simulink model "HybridVehicle"  (R2020b)
settings: Solver=ode23tb  StartTime=0.0  StopTime=1800  RelTol=1e-3
model workspace (MAT data in the model file):
  DownShiftSpeeds = [11.05  11.05  11.05  11.05  11.05  11.05  11.05  11.05  11.05  11.05  11.05  11.05  19.55  25.5  31.45  35.7  35.7; 18.7  18.7  18.7  18.7  19.125  20.48636  21.33636  23.375  27.28636  30.26136  33.827365  38.76136  46.072635  56.1  64.6  73.1  73.1; 28.9  28.9  28.9  28.9  28.9  30.51364  34.51136  41.56364  47.68636  53.377365  58.477365  65.622635  73.525  81.26136  88.48636  115.6  115.6; 38.675  38.675  38.675  38.675  39.43864  42.41364  47.68636  56.43864  65.11136  72.927365  80.497635  90.01364  100.81136  110.672635  122.4  153  153; 51.425  51.425  51.425  51.425  51.76364  55.077365  62.38864  72.422635  83.3  102  136  425  425  425  425  425  425]
  I = 0.25
  Kbr = 1000000
  MGUMaxPower = 50000
  P = 15
  PedalPositions = [0 6.2485 12.4969 18.7454 24.9939 31.2424 37.4908 43.7393 49.9878 56.2363 62.4847 68.7332 74.9817 81.2302 87.4786 93.7271 99.9756]
  SOCmax = 99
  TrqICMax = 175
  TrqMGUMax = 150
  TrqMax = 325
  UpShiftSpeeds = [12.75  12.75  12.75  12.75  12.75  12.75  15.552365  17.08636  18.7  20.227365  23.46136  27.625  31.702365  36.63636  42.5  42.5  42.5; 20.997635  20.997635  20.997635  20.997635  21.927365  24.902365  28.727365  31.78864  35.275  39.697635  46.41136  51.85  59.672635  67.48864  78.2  78.2  78.2; 31.45  31.45  31.45  31.45  34.172635  41.052365  47.175  52.952365  59.5  68  76.5  85  93.5  106.25  119.85  119.85  119.85; 42.16136  42.16136  42.16136  43.947635  47.002365  54.31364  63.325  71.227365  79.222635  88.06136  98.852365  109.052365  118.402365  128.86136  157.25  157.25  157.25; 55.58864  55.58864  55.58864  58.052365  61.53864  72.077365  85.51136  96.81364  255  255  255  255  255  255  255  255  255]
  axle_b = 10
  axle_k = 5000
  bevAxle_wc = 400
  bevNp = 2
  bevNs = 30
  brkTrqMGU = 150
  brkTrqMax = 700
  convAxle_wc = 500
  diffRatio = 3.4
  diffRatio1 = 3.4
  driveshaft_b = 10
  driveshaft_k = 2500
  driveshaft_wc = 500
  engineSpeedPoints_rpm = [750 1053.57142857 1357.14285714 1660.71428571 1964.28571429 2267.85714286 2571.42857143 2875 3178.57142857 3482.14285714 3785.71428571 4089.28571429 4392.85714286 4696.42857143 5000]
  engineTorqueMap_Nm = [-13.6738264269 15.0034460821 26.4289521305 37.8539339756 49.2854604964 60.7146317399 72.0173711595 77.7345012802 77.7345012802 77.7345012802 77.7345012802 77.7345012802 ... (240 elements, 16x15)]
  engineTorquePoints_Nm = [0 15 26.4285714286 37.8571428571 49.2857142857 60.7142857143 72.1428571429 83.5714285714 95 106.428571429 117.857142857 129.285714286 140.714285714 152.142857143 163.571428571 175]
  fuelCapacity = 35
  motorMaxTorqueNm = [500 500 500 500 500 500 416.666666667 357.142857143 312.5 277.777777778 250 227.272727273 208.333333333 192.307692308 178.571428571 166.666666667]
  motorSpeedRadPs = [0 40 80 120 160 200 240 280 320 360 400 440 480 520 560 600]
  tau_IC = 2
  tau_Regen = 1
  vehicleMass = 1500
  wheelRadius = 0.35
libraries: autolibshared x2
settings Model: Creator=ivane  LastModifiedBy=francescoprignoli
settings OptimizationCC: OptimizeBlockIOStorage=off
settings RTWCC: BuildConfiguration=Debug
settings CodeAppCC: ForceParamTrailComments=on  MATLABSourceComments=on

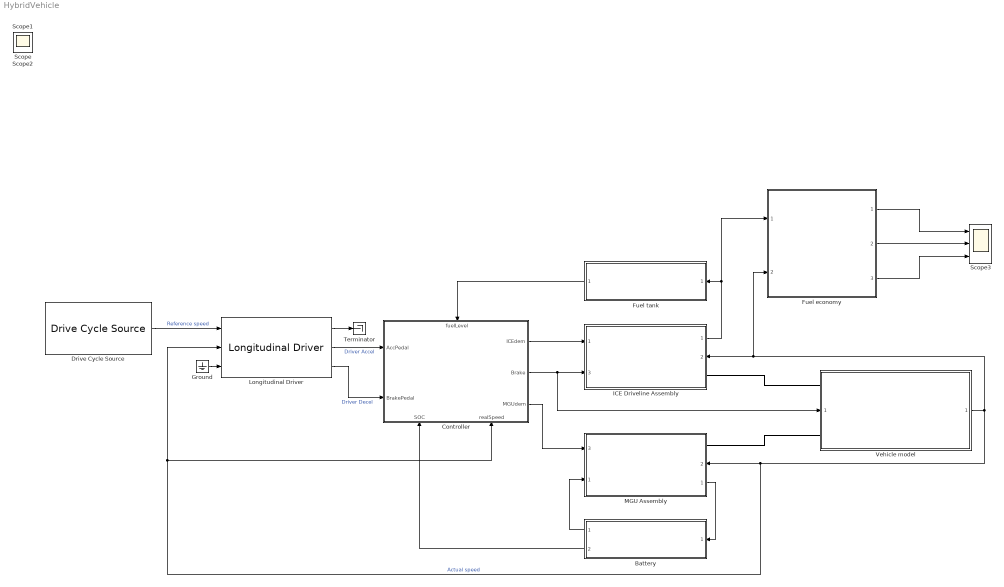
== system HybridVehicle ==
  Battery : Subsystem  ReferencedSubsystem=Battery
      settings: PortSchema="{\"entries\":[{\"content\":{\"sides\":[{\"content\":{\"connectorIds\":[\"Out1\",\"Out2\"]},\"type\":\"ConnectorPlacement.EquallySpacedRectSide\",\"uuid\":\"62c661fb-2963-4729-8409-c11ca18452bb\"},{\"content\":{\"connectorIds\":[\"In1\"],\"side\":\"RIGHT\"},\"type\":\"ConnectorPlacement.EquallySpacedRectSide\",\"uuid\":\"8d8a0df4-31a2-4844-b6e4-fdfd8750374f\"},{\"content\":{\"connectorIds\":[],\"side\":\"TOP\"},\"type\":\"ConnectorPlacement.EquallySpacedRectSide\",\"uuid\":\"345d14b7-5d59-4ed6-ba31-c78cc2155fc5\"},{\"content\":{\"connectorIds\":[],\"side\":\"HIDDEN\"},\"type\":\"ConnectorPlacement.EquallySpacedRectSide\",\"uuid\":\"be681e4d-0788-4d60-9432-78c6b7c184d6\"}]},\"type\":\"ConnectorPlacement.EquallySpacedConnector\",\"uuid\":\"76d22945-58a4-4f01-9ad4-fc5d192e1319\"}],\"packageUris\":[\"http://schema.mathworks.com/mf0/Connector/R2020b\"],\"version\":\"1.0\"}"
  Controller : Subsystem
      settings: PortSchema="{\"entries\":[{\"content\":{\"sides\":[{\"content\":{\"connectorIds\":[\"In1\",\"In2\"]},\"type\":\"ConnectorPlacement.EquallySpacedRectSide\",\"uuid\":\"9a9bdc3f-d362-44bb-99be-1b7341f9bf7a\"},{\"content\":{\"connectorIds\":[\"Out1\",\"Out2\",\"Out3\"],\"side\":\"RIGHT\"},\"type\":\"ConnectorPlacement.EquallySpacedRectSide\",\"uuid\":\"59b74d4a-d1e6-4f44-8f4c-93be4bc1758f\"},{\"content\":{\"connectorIds\":[\"In3\"],\"side\":\"TOP\"},\"type\":\"ConnectorPlacement.EquallySpacedRectSide\",\"uuid\":\"cbb51e89-e423-4cae-95cb-0d8b132c5e82\"},{\"content\":{\"connectorIds\":[\"In4\",\"In5\"],\"side\":\"BOTTOM\"},\"type\":\"ConnectorPlacement.EquallySpacedRectSide\",\"uuid\":\"125909ff-8730-4992-b334-c45829c35989\"},{\"content\":{\"connectorIds\":[],\"side\":\"HIDDEN\"},\"type\":\"ConnectorPlacement.EquallySpacedRectSide\",\"uuid\":\"e6b91313-86a6-430d-abb6-f281ee7ca3bb\"}]},\"type\":\"ConnectorPlacement.EquallySpacedConnector\",\"uuid\":\"b5413eda-bb73-4d0e-ac80-d897ae8d6098\"}],\"packageUris\":[\"http://schema.mathworks.com/mf0/Connector/R2020b\"],\"version\":\"1.0\"}"
  Drive Cycle Source : autolibshared/Drive Cycle Source  cycleVar=Workspace variable  wsVar=WLTP_class_3  fileVar=cycleFTP75.mat  tfinal="1800  seconds"  cycleRepeat=off  outAccPort=off  outGearPort=off  gearList=No gear data  t_wot1=5  xdot_woto=0  xdot_wot1=30  t_wot2=20  xdot_wot2=0  t_wotend=30  srcUnit=km/h  outUnit=km/h  srcAccUnit=m/s/s  outAccUnit=m/s^2  dt=0  aMode=1  faultOption=off  velBnd=2  velBndUnit=mph  inUnit=m/s  timeBnd=1  failOption=off  stopSim=off  maxFaultCnt=10  maxFaultTime=2  maxTotFaultTime=15  traceOption=off  dtTrace=1  traceWindow=10  lastDCname=Custom Data Set 1  lastOutUnit=mph  lastDT=0  lastTB=1  lastSB=2  forceCalcBound=off
      settings: SourceProductBaseCode=PW,MT,UV,VE,VP
  Fuel economy : Subsystem  ReferencedSubsystem=Fuel_economy
  Fuel tank : Subsystem  ReferencedSubsystem=fuelTank
  Ground : Ground
  ICE Driveline Assembly : Subsystem  ReferencedSubsystem=IC_Driveline
      settings: PortSchema="{\"entries\":[{\"content\":{\"sides\":[{\"content\":{\"connectorIds\":[\"In1\",\"In3\"]},\"type\":\"ConnectorPlacement.EquallySpacedRectSide\",\"uuid\":\"d2a2af2f-0810-46c5-a89d-1fb3bffb58b0\"},{\"content\":{\"connectorIds\":[\"Out1\",\"In2\",\"RConn1\"],\"side\":\"RIGHT\"},\"type\":\"ConnectorPlacement.EquallySpacedRectSide\",\"uuid\":\"5d91c2bd-bc93-425c-9733-5ba49e3ee9da\"},{\"content\":{\"connectorIds\":[],\"side\":\"TOP\"},\"type\":\"ConnectorPlacement.EquallySpacedRectSide\",\"uuid\":\"30272aa7-5431-486b-ba2d-786d8a62fe2e\"},{\"content\":{\"connectorIds\":[],\"side\":\"HIDDEN\"},\"type\":\"ConnectorPlacement.EquallySpacedRectSide\",\"uuid\":\"f07e1d6c-3558-4c7b-844c-ecaea33e0b73\"}]},\"type\":\"ConnectorPlacement.EquallySpacedConnector\",\"uuid\":\"e11bd347-ea62-4e54-9941-5a9032f6c7d6\"}],\"packageUris\":[\"http://schema.mathworks.com/mf0/Connector/R2020b\"],\"version\":\"1.0\"}"
  Longitudinal Driver : autolibshared/Longitudinal Driver  extAccelOvr=off  extDecelOvr=off  extAccelHld=off  extDecelHld=off  extAccelZero=off  extDecelZero=off  cntrlType=PI  shftType=None  velUnits=km/h  gearOut=off  Kp=15  Ki=0.5  Kff=0  Kg=0  VehVelVec=[0 100]  KffVec=[.1 .1]  KpVec=[10 10]  KiVec=[5 5]  KgVec=[0 0]  m=1500  Kpt=3000  tau=.1  L=2  aR=200  bR=2.5  cR=.5  g=9.81  vnom=100  Kaw=0  tauerr=.0  tauPt=2  GearInit=0  tShift=.1  pdlVec=[0.1 0.4 0.5 0.9]  upShftTbl=[-1 12.9375 26.4375 39.9375 51.18749999999999 62.4375 72.84375 83.25;-1 16.3125 29.8125 43.3125 54.5624 65.8125 76.78125 87.75;-1 19.6875 33.1875 46.68749999999999 57.9375 69.1875 80.71875 92.25;-1 33 52.5 77.25 100.5 138.75 161.875 185]  dwnShftTbl=[1 9.5625 23.0625 36.5625 47.8125 59.0625 68.90625 78.75;1 12.9375 26.4375 39.9375 51.18749999999999 62.4375 72.84375 83.25;1 16.3125 29.8125 43.3125 54.562499 65.8125 76.78125 87.75;1 19.6875 33.1875 46.68749999999999 57.9375 69.1875 80.71875 92.25]  tClutch=.5  tRev=.5  tPark=120  aMode=1  UpGearVec="[0  1  2  3  4  5  6  7]"  DownGearVec="[1  2  3  4  5  6  7  8]"
      settings: SourceProductBaseCode=PW,MT,UV,VE,VP
  MGU Assembly : Subsystem  ReferencedSubsystem=MGU
      settings: PortSchema="{\"entries\":[{\"content\":{\"sides\":[{\"content\":{\"connectorIds\":[\"In3\",\"In1\"]},\"type\":\"ConnectorPlacement.EquallySpacedRectSide\",\"uuid\":\"d2a2af2f-0810-46c5-a89d-1fb3bffb58b0\"},{\"content\":{\"connectorIds\":[\"RConn1\",\"In2\",\"Out1\"],\"side\":\"RIGHT\"},\"type\":\"ConnectorPlacement.EquallySpacedRectSide\",\"uuid\":\"5d91c2bd-bc93-425c-9733-5ba49e3ee9da\"},{\"content\":{\"connectorIds\":[],\"side\":\"TOP\"},\"type\":\"ConnectorPlacement.EquallySpacedRectSide\",\"uuid\":\"30272aa7-5431-486b-ba2d-786d8a62fe2e\"},{\"content\":{\"connectorIds\":[],\"side\":\"HIDDEN\"},\"type\":\"ConnectorPlacement.EquallySpacedRectSide\",\"uuid\":\"f07e1d6c-3558-4c7b-844c-ecaea33e0b73\"}]},\"type\":\"ConnectorPlacement.EquallySpacedConnector\",\"uuid\":\"e11bd347-ea62-4e54-9941-5a9032f6c7d6\"}],\"packageUris\":[\"http://schema.mathworks.com/mf0/Connector/R2020b\"],\"version\":\"1.0\"}"
  Scope3 : Scope  NumInputPorts=3
  Terminator : Terminator
  Vehicle model : Subsystem  ReferencedSubsystem=vehicleModel
      settings: PortSchema="{\"entries\":[{\"content\":{\"sides\":[{\"content\":{\"connectorIds\":[\"LConn1\",\"In1\",\"LConn2\"]},\"type\":\"ConnectorPlacement.EquallySpacedRectSide\",\"uuid\":\"297baffa-e0bc-4afe-8d3b-fef71b7412b4\"},{\"content\":{\"connectorIds\":[\"Out1\"],\"side\":\"RIGHT\"},\"type\":\"ConnectorPlacement.EquallySpacedRectSide\",\"uuid\":\"8a12a35b-b522-4ba0-9ba0-852b497f573e\"},{\"content\":{\"connectorIds\":[],\"side\":\"TOP\"},\"type\":\"ConnectorPlacement.EquallySpacedRectSide\",\"uuid\":\"b4b51f6d-39af-472b-beff-f9410fe777e8\"},{\"content\":{\"connectorIds\":[],\"side\":\"HIDDEN\"},\"type\":\"ConnectorPlacement.EquallySpacedRectSide\",\"uuid\":\"ccc4846e-18b0-46b1-8b77-dbf40ce11e43\"}]},\"type\":\"ConnectorPlacement.EquallySpacedConnector\",\"uuid\":\"224bfd92-7422-4b82-8ee3-7d4031b335e8\"}],\"packageUris\":[\"http://schema.mathworks.com/mf0/Connector/R2020b\"],\"version\":\"1.0\"}"
  Scope : Scope
  Scope1 : Scope
  Scope2 : Scope
  wires:
  Longitudinal Driver/2 -> Controller/1(AccPedal)  "Driver Accel"
  Longitudinal Driver/3 -> Controller/2(BrakePedal)  "Driver Decel"
  Controller/1(ICEdem) -> ICE Driveline Assembly/1
  Controller/2(Brake) -> Vehicle model/1, ICE Driveline Assembly/3
  Fuel tank/1 -> Controller/3(fuelLevel)
  ICE Driveline Assembly/1 -> Fuel economy/1, Fuel tank/1
  Controller/3(MGUdem) -> MGU Assembly/3
  MGU Assembly/1 -> Battery/1
  Battery/1 -> MGU Assembly/1
  Battery/2 -> Controller/4(SOC)
  Vehicle model/1 -> Fuel economy/2, ICE Driveline Assembly/2, MGU Assembly/2, Longitudinal Driver/2, Controller/5(realSpeed)  "Actual speed"
  Drive Cycle Source/1 -> Longitudinal Driver/1  "Reference speed"
  Ground/1 -> Longitudinal Driver/3
  Longitudinal Driver/1 -> Terminator/1
  Fuel economy/3 -> Scope3/3
  Fuel economy/1 -> Scope3/1
  Fuel economy/2 -> Scope3/2
  connections:
  ICE Driveline Assembly/RConn1 -- Vehicle model/LConn1
  Vehicle model/LConn2 -- MGU Assembly/RConn1

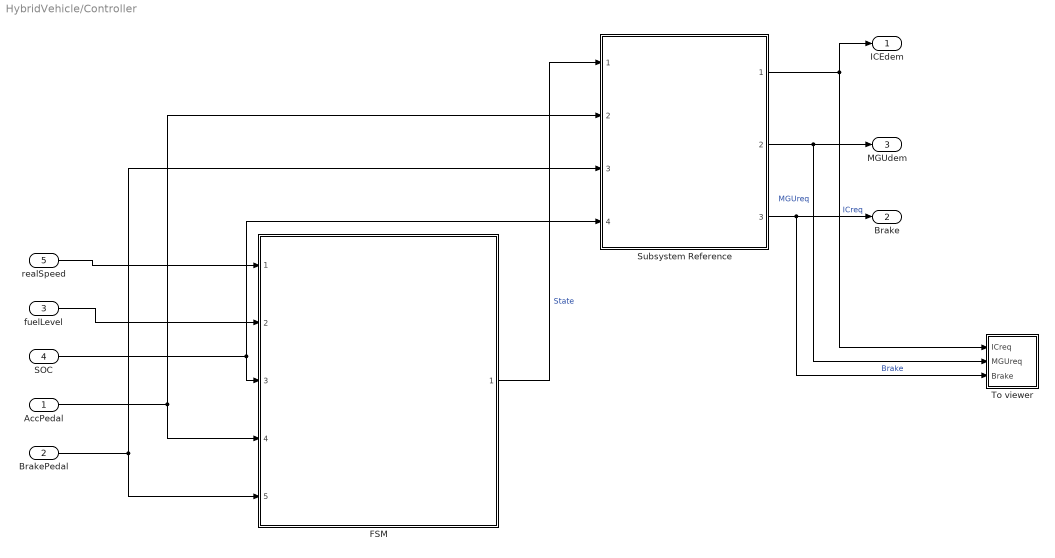
== system HybridVehicle/Controller ==
  AccPedal : Inport
  BrakePedal : Inport  Port=2
  fuelLevel : Inport  Port=3
  SOC : Inport  Port=4
  realSpeed : Inport  Port=5
  FSM : Subsystem  ReferencedSubsystem=stateMachine
  Subsystem Reference : Subsystem  ReferencedSubsystem=TrqDemController
  To viewer : Subsystem
  ICEdem : Outport
  Brake : Outport  Port=2
  MGUdem : Outport  Port=3
  wires:
  AccPedal/1 -> Subsystem Reference/2, FSM/4
  BrakePedal/1 -> Subsystem Reference/3, FSM/5
  SOC/1 -> Subsystem Reference/4, FSM/3
  fuelLevel/1 -> FSM/2
  realSpeed/1 -> FSM/1
  Subsystem Reference/1 -> To viewer/1(ICreq), ICEdem/1  "ICreq"
  Subsystem Reference/2 -> To viewer/2(MGUreq), MGUdem/1  "MGUreq"
  Subsystem Reference/3 -> To viewer/3(Brake), Brake/1  "Brake"
  FSM/1 -> Subsystem Reference/1  "State"

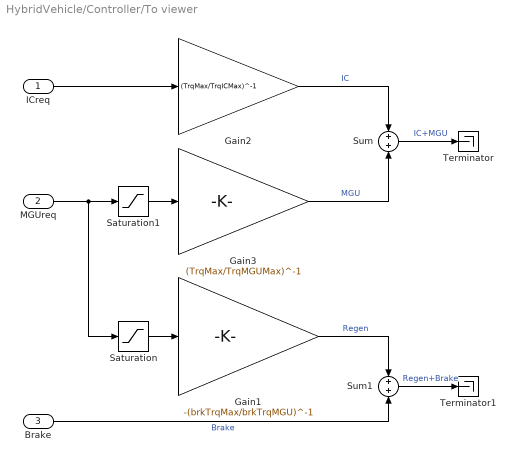
== system HybridVehicle/Controller/To viewer ==
  ICreq : Inport
  MGUreq : Inport  Port=2
  Brake : Inport  Port=3
  Gain1 : Gain  Gain=-(brkTrqMax/brkTrqMGU)^-1
  Gain2 : Gain  Gain=(TrqMax/TrqICMax)^-1
  Gain3 : Gain  Gain=(TrqMax/TrqMGUMax)^-1
  Saturation : Saturate  UpperLimit=0  LowerLimit=-1
  Saturation1 : Saturate  UpperLimit=1  LowerLimit=0
  Sum : Sum  Inputs=+|+
  Sum1 : Sum  Inputs=+|+
  Terminator : Terminator
  Terminator1 : Terminator
  wires:
  Sum1/1 -> Terminator1/1  "Regen+Brake"
  MGUreq/1 -> Saturation/1, Saturation1/1
  Gain3/1 -> Sum/2  "MGU"
  Gain2/1 -> Sum/1  "IC"
  Brake/1 -> Sum1/2  "Brake"
  ICreq/1 -> Gain2/1
  Gain1/1 -> Sum1/1  "Regen"
  Sum/1 -> Terminator/1  "IC+MGU"
  Saturation/1 -> Gain1/1
  Saturation1/1 -> Gain3/1
